simulink model "SecRwRtStBkReclnTrgtPosSelc"  (R2018b)
settings: Solver=FixedStepDiscrete  StartTime=0.0  StopTime=10.0  FixedStep=0.01  RelTol=1e-3
undefined symbols (not defined in the file or in its folder): KeSMSw4SAcsMd23SecRwRtStBkReclnUpwdDnwdPos_Val, KeSMSw4SAcsMd23SecRwRtStBkReclnUpwdDnwdPosMax_Val, KeSMSw4SAcsMd23SecRwRtStBkReclnUpwdDnwdPosMin_Val, KeSMSw4SAcsMd24SecRwRtStBkReclnUpwdDnwdPos1_Val, KeSMSw4SAcsMd24SecRwRtStBkReclnUpwdDnwdPos2_Val, KeSMSw4SAcsMd24SecRwRtStBkReclnUpwdDnwdPosMax1_Val, KeSMSw4SAcsMd24SecRwRtStBkReclnUpwdDnwdPosMax2_Val, KeSMSw4SAcsMd24SecRwRtStBkReclnUpwdDnwdPosMin1_Val, KeSMSw4SAcsMd24SecRwRtStBkReclnUpwdDnwdPosMin2_Val, KeSMSw4SAcsMd25SecRwRtStBkReclnUpwdDnwdPos_Val, KeSMSw4SAcsMd25SecRwRtStBkReclnUpwdDnwdPosMax_Val, KeSMSw4SAcsMd25SecRwRtStBkReclnUpwdDnwdPosMin_Val, KeSMSw4SAcsMd26SecRwRtStBkReclnUpwdDnwdPos_Val, KeSMSw4SAcsMd26SecRwRtStBkReclnUpwdDnwdPosMax_Val, KeSMSw4SAcsMd26SecRwRtStBkReclnUpwdDnwdPosMin_Val, KeSMSw4sLyingMDSecRwRtStBkReclnUpwdDnwdPos_Val, KeSMSw4sLyingMDSecRwRtStBkReclnUpwdDnwdPosMax_Val, KeSMSw4sLyingMDSecRwRtStBkReclnUpwdDnwdPosMin_Val, KeSMSw4sRecoveryMDSecRwRtStBkReclnUpwdDnwdPos_Val, KeSMSw4sRecoveryMDSecRwRtStBkReclnUpwdDnwdPosMax_Val, KeSMSw4sRecoveryMDSecRwRtStBkReclnUpwdDnwdPosMin_Val, KeSMSw4sVIPMDSecRwRtStBkReclnUpwdDnwdPos_Val, KeSMSw4sVIPMDSecRwRtStBkReclnUpwdDnwdPosMax_Val, KeSMSw4sVIPMDSecRwRtStBkReclnUpwdDnwdPosMin_Val, KeSMSw6sAcsEntrySecRwRtStBkReclnUpwdDnwd1Pos_Val, KeSMSw6sAcsEntrySecRwRtStBkReclnUpwdDnwdPos1Max_Val, KeSMSw6sAcsEntrySecRwRtStBkReclnUpwdDnwdPos1Min_Val, KeSMSw6sAcsEntrySecRwRtStBkReclnUpwdDnwdPos_Val, KeSMSw6sAcsEntrySecRwRtStBkReclnUpwdDnwdPosMax_Val, KeSMSw6sAcsEntrySecRwRtStBkReclnUpwdDnwdPosMin_Val, KeSMSw6sAcsExtSecRwRtStBkReclnUpwdDnwdPos_Val, KeSMSw6sAcsExtSecRwRtStBkReclnUpwdDnwdPosMax_Val, KeSMSw6sAcsExtSecRwRtStBkReclnUpwdDnwdPosMin_Val, KeSMSw6sRecoveryMdSecRwRtStBkReclnUpwdDnwdPos_Val, KeSMSw6sRecoveryMdSecRwRtStBkReclnUpwdDnwdPosMax_Val, KeSMSw6sRecoveryMdSecRwRtStBkReclnUpwdDnwdPosMin_Val, KeSMSw6sVIPSecRwRtStBkReclnUpwdDnwdPos_Val, KeSMSw6sVIPSecRwRtStBkReclnUpwdDnwdPosMax_Val, KeSMSw6sVIPSecRwRtStBkReclnUpwdDnwdPosMin_Val, KeSMSwAcsEntrySecRwRtStBkReclnUpwdDnwdPos1_Val, KeSMSwAcsEntrySecRwRtStBkReclnUpwdDnwdPos1Max_Val, KeSMSwAcsEntrySecRwRtStBkReclnUpwdDnwdPos1Min_Val, KeSMSwAcsEntrySecRwRtStBkReclnUpwdDnwdPos_Val, KeSMSwAcsEntrySecRwRtStBkReclnUpwdDnwdPosMax_Val, KeSMSwAcsEntrySecRwRtStBkReclnUpwdDnwdPosMin_Val, KeSMSwAcsExtSecRwRtStBkReclnUpwdDnwdPos_Val, KeSMSwAcsExtSecRwRtStBkReclnUpwdDnwdPosMax_Val, KeSMSwAcsExtSecRwRtStBkReclnUpwdDnwdPosMin_Val, KeSMSwAcsMd32SecRwRtStBkReclnUpwdDnwdPos1_Val, KeSMSwAcsMd32SecRwRtStBkReclnUpwdDnwdPos1Max_Val, KeSMSwAcsMd32SecRwRtStBkReclnUpwdDnwdPos1Min_Val, KeSMSwAcsMd32SecRwRtStBkReclnUpwdDnwdPos_Val, KeSMSwAcsMd32SecRwRtStBkReclnUpwdDnwdPosMax_Val, KeSMSwAcsMd32SecRwRtStBkReclnUpwdDnwdPosMin_Val, KeSMSwAcsMd53SecRwRtStBkReclnUpwdDnwdPos1_Val, KeSMSwAcsMd53SecRwRtStBkReclnUpwdDnwdPos1Max_Val, KeSMSwAcsMd53SecRwRtStBkReclnUpwdDnwdPos1Min_Val, KeSMSwAcsMd53SecRwRtStBkReclnUpwdDnwdPos_Val, KeSMSwAcsMd53SecRwRtStBkReclnUpwdDnwdPosMax_Val, KeSMSwAcsMd53SecRwRtStBkReclnUpwdDnwdPosMin_Val ... (+12)
libraries: TrgtPosSelcLib x15, simulink x2
(part 1 of 2)
settings Model: Creator=sn2xws  LastModifiedBy=sn2xws
settings Model: ModifiedHistory=|
  | 2023.8.1 V2.0.0 CR421790 增加模式21-26
  | 2023.11.7 bug 554442 便利下车max min 标定改为两套
  | 2024.5.7 V3.0.0 557 eze模式变更
  | 2024.7.8 V3.0.1 557模式流程V1.9
  | 2024.8.16 V3.0.2 靠背标定选择模块修改MD8 MD9逻辑
  | 2024 8.17 V3.0.3 md1 靠背阶段1阶段2目标位置选择逻辑变更
  | 2024.8.20 V3.0.4 md32 md53靠背选择改用CushnPos判断
settings DataIOCC: SaveFormat=StructureWithTime
settings OptimizationCC: DefaultParameterBehavior=Inlined  EnhancedBackFolding=on  PassReuseOutputArgsAs=Individual arguments  ZeroExternalMemoryAtStartup=off  ZeroInternalMemoryAtStartup=off  OptimizeBlockOrder=speed  DifferentSizesBufferReuse=on  OptimizationCustomize=off
settings DebuggingCC: ParameterTunabilityLossMsg=error
settings SFSimCC: MATLABDynamicMemAlloc=off
settings RTWCC: SystemTargetFile=autosar.tlc  GenCodeOnly=on  TemplateMakefile=ert_default_tmf  Description=AUTOSAR  GenerateReport=on  IncludeHyperlinkInReport=on  LaunchReport=on  GenerateTraceInfo=on  GenerateTraceReport=on  GenerateTraceReportSl=on  GenerateTraceReportSf=on  GenerateTraceReportEml=on  GenerateCodeMetricsReport=on
settings CodeAppCC: ForceParamTrailComments=on  IgnoreCustomStorageClasses=off  OperatorAnnotations=on  SimulinkDataObjDesc=on  SFDataObjDesc=on  InsertBlockDesc=on
settings STFCustomTargetCC: TargetLangStandard=C99 (ISO)  MultiwordLength=256  ParMdlRefBuildCompliant=on  CompOptLevelCompliant=on  IncludeMdlTerminateFcn=off  CombineOutputUpdateFcns=on  SuppressErrorStatus=on  ERTCustomFileBanners=on  SupportNonFinite=off  SupportComplex=off  SupportContinuousTime=off  SupportNonInlinedSFcns=off  RemoveResetFunc=on  MATLABClassNameForMDSCustomization=Simulink.SoftwareTarget.ERTCustomization  AutosarCompliant=on  UseToolchainInfoCompliant=on  LookupTableObjectStructAxisOrder=2,1,3,4,...  LUTObjectStructOrderEvenSpacing=Size,Table,Breakpoints  SystemTargetFile=autosar.tlc
settings ERTTargetCC: TargetLangStandard=C99 (ISO)  ConcurrentExecutionCompliant=off  IncludeMdlTerminateFcn=off  SuppressErrorStatus=on  SupportNonFinite=off  SupportComplex=off  ModelStepFunctionPrototypeControlCompliant=off  CPPClassGenCompliant=off  AutosarCompliant=on  LookupTableObjectStructAxisOrder=2,1,3,4,...  LUTObjectStructOrderEvenSpacing=Size,Table,Breakpoints  InlinedParameterPlacement=NonHierarchical  ERTCustomFileTemplate=example_file_process.tlc  ERTFilePackagingFormat=Compact

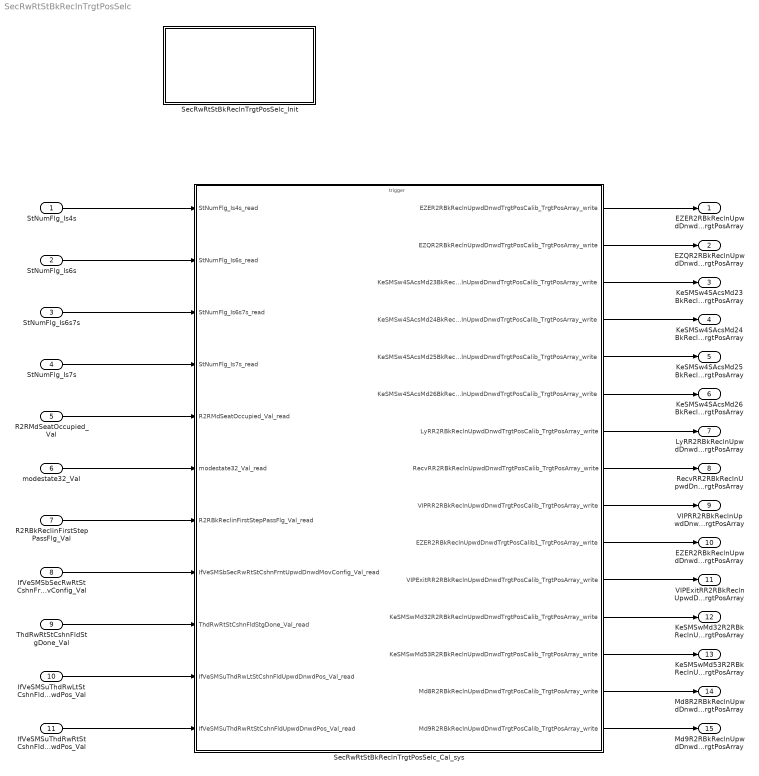
== system SecRwRtStBkReclnTrgtPosSelc ==
  StNumFlg_Is4s : Inport  OutDataTypeStr=boolean  PortDimensions=1
  StNumFlg_Is6s : Inport  Port=2  OutDataTypeStr=boolean  PortDimensions=1
  StNumFlg_Is6s7s : Inport  Port=3  OutDataTypeStr=boolean  PortDimensions=1
  StNumFlg_Is7s : Inport  Port=4  OutDataTypeStr=boolean  PortDimensions=1
  R2RMdSeatOccupied_Val : Inport  Port=5  OutDataTypeStr=boolean  PortDimensions=1
  modestate32_Val : Inport  Port=6  OutDataTypeStr=uint32  PortDimensions=1
  R2RBkReclinFirstStepPassFlg_Val : Inport  Port=7  OutDataTypeStr=boolean  PortDimensions=1
  IfVeSMSbSecRwRtStCshnFrntUpwdDnwdMovConfig_Val : Inport  Port=8  OutDataTypeStr=boolean  PortDimensions=1
  ThdRwRtStCshnFldStgDone_Val : Inport  Port=9  OutDataTypeStr=boolean  PortDimensions=1
  IfVeSMSuThdRwLtStCshnFldUpwdDnwdPos_Val : Inport  Port=10  OutDataTypeStr=uint16  PortDimensions=1
  IfVeSMSuThdRwRtStCshnFldUpwdDnwdPos_Val : Inport  Port=11  OutDataTypeStr=uint16  PortDimensions=1
  SecRwRtStBkReclnTrgtPosSelc_Cal_sys : Subsystem
  SecRwRtStBkReclnTrgtPosSelc_Init : Subsystem
  EZER2RBkReclnUpwdDnwdTrgtPosCalib_TrgtPosArray : Outport  Description=|  OutDataTypeStr=uint16  PortDimensions=3
      | 0:Pos
      | 1:Max
      | 2:Min
  EZQR2RBkReclnUpwdDnwdTrgtPosCalib_TrgtPosArray : Outport  Description=|  Port=2  OutDataTypeStr=uint16  PortDimensions=3
      | 0:Pos
      | 1:Max
      | 2:Min
  KeSMSw4SAcsMd23BkReclnUpwdDnwdTrgtPosCalib_TrgtPosArray : Outport  Description=|  Port=3  OutDataTypeStr=uint16  PortDimensions=3
      | 0:Pos
      | 1:Max
      | 2:Min
  KeSMSw4SAcsMd24BkReclnUpwdDnwdTrgtPosCalib_TrgtPosArray : Outport  Description=|  Port=4  OutDataTypeStr=uint16  PortDimensions=3
      | 0:Pos
      | 1:Max
      | 2:Min
  KeSMSw4SAcsMd25BkReclnUpwdDnwdTrgtPosCalib_TrgtPosArray : Outport  Description=|  Port=5  OutDataTypeStr=uint16  PortDimensions=3
      | 0:Pos
      | 1:Max
      | 2:Min
  KeSMSw4SAcsMd26BkReclnUpwdDnwdTrgtPosCalib_TrgtPosArray : Outport  Description=|  Port=6  OutDataTypeStr=uint16  PortDimensions=3
      | 0:Pos
      | 1:Max
      | 2:Min
  LyRR2RBkReclnUpwdDnwdTrgtPosCalib_TrgtPosArray : Outport  Description=|  Port=7  OutDataTypeStr=uint16  PortDimensions=3
      | 0:Pos
      | 1:Max
      | 2:Min
  RecvRR2RBkReclnUpwdDnwdTrgtPosCalib_TrgtPosArray : Outport  Description=|  Port=8  OutDataTypeStr=uint16  PortDimensions=3
      | 0:Pos
      | 1:Max
      | 2:Min
  VIPRR2RBkReclnUpwdDnwdTrgtPosCalib_TrgtPosArray : Outport  Description=|  Port=9  OutDataTypeStr=uint16  PortDimensions=3
      | 0:Pos
      | 1:Max
      | 2:Min
  EZER2RBkReclnUpwdDnwdTrgtPosCalib1_TrgtPosArray : Outport  Description=|  Port=10  OutDataTypeStr=uint16  PortDimensions=3
      | 0:Pos
      | 1:Max
      | 2:Min
  VIPExitRR2RBkReclnUpwdDnwdTrgtPosCalib_TrgtPosArray : Outport  Description=|  Port=11  OutDataTypeStr=uint16  PortDimensions=3
      | 0:Pos
      | 1:Max
      | 2:Min
  KeSMSwMd32R2RBkReclnUpwdDnwdTrgtPosCalib_TrgtPosArray : Outport  Description=|  Port=12  OutDataTypeStr=uint16  PortDimensions=3
      | 0:Pos
      | 1:Max
      | 2:Min
  KeSMSwMd53R2RBkReclnUpwdDnwdTrgtPosCalib_TrgtPosArray : Outport  Description=|  Port=13  OutDataTypeStr=uint16  PortDimensions=3
      | 0:Pos
      | 1:Max
      | 2:Min
  Md8R2RBkReclnUpwdDnwdTrgtPosCalib_TrgtPosArray : Outport  Description=|  Port=14  OutDataTypeStr=uint16  PortDimensions=3
      | 0:Pos
      | 1:Max
      | 2:Min
  Md9R2RBkReclnUpwdDnwdTrgtPosCalib_TrgtPosArray : Outport  Description=|  Port=15  OutDataTypeStr=uint16  PortDimensions=3
      | 0:Pos
      | 1:Max
      | 2:Min
  wires:
  StNumFlg_Is4s/1 -> SecRwRtStBkReclnTrgtPosSelc_Cal_sys/1(StNumFlg_Is4s_read)
  StNumFlg_Is6s/1 -> SecRwRtStBkReclnTrgtPosSelc_Cal_sys/2(StNumFlg_Is6s_read)
  StNumFlg_Is6s7s/1 -> SecRwRtStBkReclnTrgtPosSelc_Cal_sys/3(StNumFlg_Is6s7s_read)
  StNumFlg_Is7s/1 -> SecRwRtStBkReclnTrgtPosSelc_Cal_sys/4(StNumFlg_Is7s_read)
  SecRwRtStBkReclnTrgtPosSelc_Cal_sys/1(EZER2RBkReclnUpwdDnwdTrgtPosCalib_TrgtPosArray_write) -> EZER2RBkReclnUpwdDnwdTrgtPosCalib_TrgtPosArray/1
  SecRwRtStBkReclnTrgtPosSelc_Cal_sys/2(EZQR2RBkReclnUpwdDnwdTrgtPosCalib_TrgtPosArray_write) -> EZQR2RBkReclnUpwdDnwdTrgtPosCalib_TrgtPosArray/1
  SecRwRtStBkReclnTrgtPosSelc_Cal_sys/3(KeSMSw4SAcsMd23BkReclnUpwdDnwdTrgtPosCalib_TrgtPosArray_write) -> KeSMSw4SAcsMd23BkReclnUpwdDnwdTrgtPosCalib_TrgtPosArray/1
  SecRwRtStBkReclnTrgtPosSelc_Cal_sys/4(KeSMSw4SAcsMd24BkReclnUpwdDnwdTrgtPosCalib_TrgtPosArray_write) -> KeSMSw4SAcsMd24BkReclnUpwdDnwdTrgtPosCalib_TrgtPosArray/1
  SecRwRtStBkReclnTrgtPosSelc_Cal_sys/5(KeSMSw4SAcsMd25BkReclnUpwdDnwdTrgtPosCalib_TrgtPosArray_write) -> KeSMSw4SAcsMd25BkReclnUpwdDnwdTrgtPosCalib_TrgtPosArray/1
  SecRwRtStBkReclnTrgtPosSelc_Cal_sys/6(KeSMSw4SAcsMd26BkReclnUpwdDnwdTrgtPosCalib_TrgtPosArray_write) -> KeSMSw4SAcsMd26BkReclnUpwdDnwdTrgtPosCalib_TrgtPosArray/1
  SecRwRtStBkReclnTrgtPosSelc_Cal_sys/7(LyRR2RBkReclnUpwdDnwdTrgtPosCalib_TrgtPosArray_write) -> LyRR2RBkReclnUpwdDnwdTrgtPosCalib_TrgtPosArray/1
  SecRwRtStBkReclnTrgtPosSelc_Cal_sys/8(RecvRR2RBkReclnUpwdDnwdTrgtPosCalib_TrgtPosArray_write) -> RecvRR2RBkReclnUpwdDnwdTrgtPosCalib_TrgtPosArray/1
  SecRwRtStBkReclnTrgtPosSelc_Cal_sys/9(VIPRR2RBkReclnUpwdDnwdTrgtPosCalib_TrgtPosArray_write) -> VIPRR2RBkReclnUpwdDnwdTrgtPosCalib_TrgtPosArray/1
  R2RMdSeatOccupied_Val/1 -> SecRwRtStBkReclnTrgtPosSelc_Cal_sys/5(R2RMdSeatOccupied_Val_read)
  modestate32_Val/1 -> SecRwRtStBkReclnTrgtPosSelc_Cal_sys/6(modestate32_Val_read)
  R2RBkReclinFirstStepPassFlg_Val/1 -> SecRwRtStBkReclnTrgtPosSelc_Cal_sys/7(R2RBkReclinFirstStepPassFlg_Val_read)
  SecRwRtStBkReclnTrgtPosSelc_Cal_sys/10(EZER2RBkReclnUpwdDnwdTrgtPosCalib1_TrgtPosArray_write) -> EZER2RBkReclnUpwdDnwdTrgtPosCalib1_TrgtPosArray/1
  IfVeSMSbSecRwRtStCshnFrntUpwdDnwdMovConfig_Val/1 -> SecRwRtStBkReclnTrgtPosSelc_Cal_sys/8(IfVeSMSbSecRwRtStCshnFrntUpwdDnwdMovConfig_Val_read)
  SecRwRtStBkReclnTrgtPosSelc_Cal_sys/11(VIPExitRR2RBkReclnUpwdDnwdTrgtPosCalib_TrgtPosArray_write) -> VIPExitRR2RBkReclnUpwdDnwdTrgtPosCalib_TrgtPosArray/1
  ThdRwRtStCshnFldStgDone_Val/1 -> SecRwRtStBkReclnTrgtPosSelc_Cal_sys/9(ThdRwRtStCshnFldStgDone_Val_read)
  SecRwRtStBkReclnTrgtPosSelc_Cal_sys/12(KeSMSwMd32R2RBkReclnUpwdDnwdTrgtPosCalib_TrgtPosArray_write) -> KeSMSwMd32R2RBkReclnUpwdDnwdTrgtPosCalib_TrgtPosArray/1
  SecRwRtStBkReclnTrgtPosSelc_Cal_sys/13(KeSMSwMd53R2RBkReclnUpwdDnwdTrgtPosCalib_TrgtPosArray_write) -> KeSMSwMd53R2RBkReclnUpwdDnwdTrgtPosCalib_TrgtPosArray/1
  SecRwRtStBkReclnTrgtPosSelc_Cal_sys/14(Md8R2RBkReclnUpwdDnwdTrgtPosCalib_TrgtPosArray_write) -> Md8R2RBkReclnUpwdDnwdTrgtPosCalib_TrgtPosArray/1
  SecRwRtStBkReclnTrgtPosSelc_Cal_sys/15(Md9R2RBkReclnUpwdDnwdTrgtPosCalib_TrgtPosArray_write) -> Md9R2RBkReclnUpwdDnwdTrgtPosCalib_TrgtPosArray/1
  IfVeSMSuThdRwLtStCshnFldUpwdDnwdPos_Val/1 -> SecRwRtStBkReclnTrgtPosSelc_Cal_sys/10(IfVeSMSuThdRwLtStCshnFldUpwdDnwdPos_Val_read)
  IfVeSMSuThdRwRtStCshnFldUpwdDnwdPos_Val/1 -> SecRwRtStBkReclnTrgtPosSelc_Cal_sys/11(IfVeSMSuThdRwRtStCshnFldUpwdDnwdPos_Val_read)

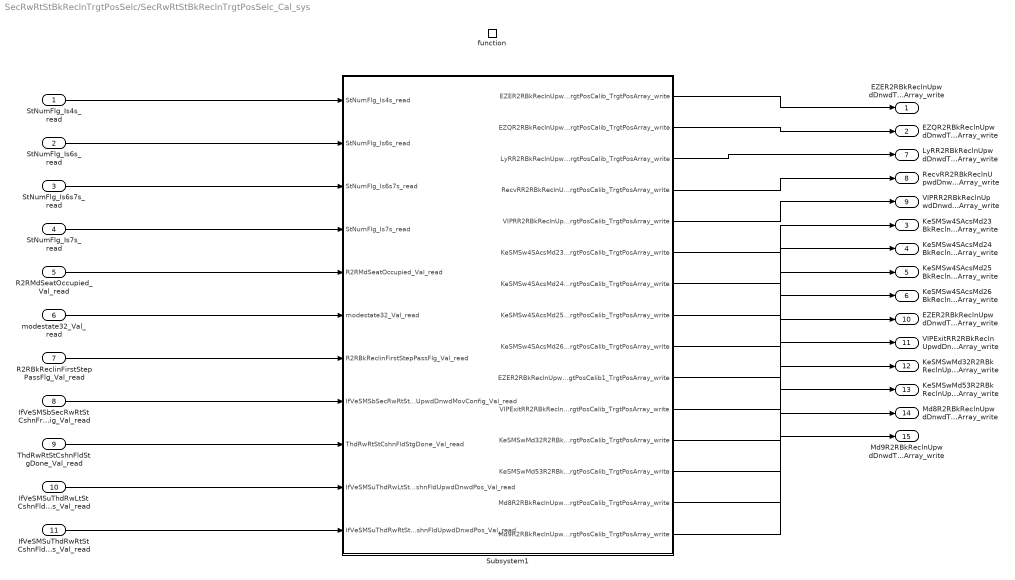
== system SecRwRtStBkReclnTrgtPosSelc/SecRwRtStBkReclnTrgtPosSelc_Cal_sys ==
  StNumFlg_Is4s_read : Inport
  StNumFlg_Is6s_read : Inport  Port=2
  StNumFlg_Is6s7s_read : Inport  Port=3
  StNumFlg_Is7s_read : Inport  Port=4
  R2RMdSeatOccupied_Val_read : Inport  Port=5
  modestate32_Val_read : Inport  Port=6
  R2RBkReclinFirstStepPassFlg_Val_read : Inport  Port=7
  IfVeSMSbSecRwRtStCshnFrntUpwdDnwdMovConfig_Val_read : Inport  Port=8
  ThdRwRtStCshnFldStgDone_Val_read : Inport  Port=9
  IfVeSMSuThdRwLtStCshnFldUpwdDnwdPos_Val_read : Inport  Port=10
  IfVeSMSuThdRwRtStCshnFldUpwdDnwdPos_Val_read : Inport  Port=11
  function : TriggerPort  TriggerType=function-call  IsSimulinkFunction=on  FunctionName=SecRwRtStBkReclnTrgtPosSelc_Cal  VariantControl=(inherit)
  Subsystem1 : Subsystem
  EZER2RBkReclnUpwdDnwdTrgtPosCalib_TrgtPosArray_write : Outport
      settings: EnsureOutportIsVirtual=on
  EZQR2RBkReclnUpwdDnwdTrgtPosCalib_TrgtPosArray_write : Outport  Port=2
      settings: EnsureOutportIsVirtual=on
  KeSMSw4SAcsMd23BkReclnUpwdDnwdTrgtPosCalib_TrgtPosArray_write : Outport  Port=3
      settings: EnsureOutportIsVirtual=on
  KeSMSw4SAcsMd24BkReclnUpwdDnwdTrgtPosCalib_TrgtPosArray_write : Outport  Port=4
      settings: EnsureOutportIsVirtual=on
  KeSMSw4SAcsMd25BkReclnUpwdDnwdTrgtPosCalib_TrgtPosArray_write : Outport  Port=5
      settings: EnsureOutportIsVirtual=on
  KeSMSw4SAcsMd26BkReclnUpwdDnwdTrgtPosCalib_TrgtPosArray_write : Outport  Port=6
      settings: EnsureOutportIsVirtual=on
  LyRR2RBkReclnUpwdDnwdTrgtPosCalib_TrgtPosArray_write : Outport  Port=7
      settings: EnsureOutportIsVirtual=on
  RecvRR2RBkReclnUpwdDnwdTrgtPosCalib_TrgtPosArray_write : Outport  Port=8
      settings: EnsureOutportIsVirtual=on
  VIPRR2RBkReclnUpwdDnwdTrgtPosCalib_TrgtPosArray_write : Outport  Port=9
      settings: EnsureOutportIsVirtual=on
  EZER2RBkReclnUpwdDnwdTrgtPosCalib1_TrgtPosArray_write : Outport  Port=10
      settings: EnsureOutportIsVirtual=on
  VIPExitRR2RBkReclnUpwdDnwdTrgtPosCalib_TrgtPosArray_write : Outport  Port=11
      settings: EnsureOutportIsVirtual=on
  KeSMSwMd32R2RBkReclnUpwdDnwdTrgtPosCalib_TrgtPosArray_write : Outport  Port=12
      settings: EnsureOutportIsVirtual=on
  KeSMSwMd53R2RBkReclnUpwdDnwdTrgtPosCalib_TrgtPosArray_write : Outport  Port=13
      settings: EnsureOutportIsVirtual=on
  Md8R2RBkReclnUpwdDnwdTrgtPosCalib_TrgtPosArray_write : Outport  Port=14
      settings: EnsureOutportIsVirtual=on
  Md9R2RBkReclnUpwdDnwdTrgtPosCalib_TrgtPosArray_write : Outport  Port=15
      settings: EnsureOutportIsVirtual=on
  wires:
  Subsystem1/3(LyRR2RBkReclnUpwdDnwdTrgtPosCalib_TrgtPosArray_write) -> LyRR2RBkReclnUpwdDnwdTrgtPosCalib_TrgtPosArray_write/1
  Subsystem1/4(RecvRR2RBkReclnUpwdDnwdTrgtPosCalib_TrgtPosArray_write) -> RecvRR2RBkReclnUpwdDnwdTrgtPosCalib_TrgtPosArray_write/1
  Subsystem1/7(KeSMSw4SAcsMd24BkReclnUpwdDnwdTrgtPosCalib_TrgtPosArray_write) -> KeSMSw4SAcsMd24BkReclnUpwdDnwdTrgtPosCalib_TrgtPosArray_write/1
  Subsystem1/8(KeSMSw4SAcsMd25BkReclnUpwdDnwdTrgtPosCalib_TrgtPosArray_write) -> KeSMSw4SAcsMd25BkReclnUpwdDnwdTrgtPosCalib_TrgtPosArray_write/1
  Subsystem1/1(EZER2RBkReclnUpwdDnwdTrgtPosCalib_TrgtPosArray_write) -> EZER2RBkReclnUpwdDnwdTrgtPosCalib_TrgtPosArray_write/1
  Subsystem1/2(EZQR2RBkReclnUpwdDnwdTrgtPosCalib_TrgtPosArray_write) -> EZQR2RBkReclnUpwdDnwdTrgtPosCalib_TrgtPosArray_write/1
  Subsystem1/5(VIPRR2RBkReclnUpwdDnwdTrgtPosCalib_TrgtPosArray_write) -> VIPRR2RBkReclnUpwdDnwdTrgtPosCalib_TrgtPosArray_write/1
  Subsystem1/6(KeSMSw4SAcsMd23BkReclnUpwdDnwdTrgtPosCalib_TrgtPosArray_write) -> KeSMSw4SAcsMd23BkReclnUpwdDnwdTrgtPosCalib_TrgtPosArray_write/1
  Subsystem1/9(KeSMSw4SAcsMd26BkReclnUpwdDnwdTrgtPosCalib_TrgtPosArray_write) -> KeSMSw4SAcsMd26BkReclnUpwdDnwdTrgtPosCalib_TrgtPosArray_write/1
  StNumFlg_Is4s_read/1 -> Subsystem1/1(StNumFlg_Is4s_read)
  StNumFlg_Is6s_read/1 -> Subsystem1/2(StNumFlg_Is6s_read)
  StNumFlg_Is6s7s_read/1 -> Subsystem1/3(StNumFlg_Is6s7s_read)
  StNumFlg_Is7s_read/1 -> Subsystem1/4(StNumFlg_Is7s_read)
  R2RMdSeatOccupied_Val_read/1 -> Subsystem1/5(R2RMdSeatOccupied_Val_read)
  Subsystem1/10(EZER2RBkReclnUpwdDnwdTrgtPosCalib1_TrgtPosArray_write) -> EZER2RBkReclnUpwdDnwdTrgtPosCalib1_TrgtPosArray_write/1
  modestate32_Val_read/1 -> Subsystem1/6(modestate32_Val_read)
  R2RBkReclinFirstStepPassFlg_Val_read/1 -> Subsystem1/7(R2RBkReclinFirstStepPassFlg_Val_read)
  Subsystem1/11(VIPExitRR2RBkReclnUpwdDnwdTrgtPosCalib_TrgtPosArray_write) -> VIPExitRR2RBkReclnUpwdDnwdTrgtPosCalib_TrgtPosArray_write/1
  IfVeSMSbSecRwRtStCshnFrntUpwdDnwdMovConfig_Val_read/1 -> Subsystem1/8(IfVeSMSbSecRwRtStCshnFrntUpwdDnwdMovConfig_Val_read)
  Subsystem1/13(KeSMSwMd53R2RBkReclnUpwdDnwdTrgtPosCalib_TrgtPosArray_write) -> KeSMSwMd53R2RBkReclnUpwdDnwdTrgtPosCalib_TrgtPosArray_write/1
  ThdRwRtStCshnFldStgDone_Val_read/1 -> Subsystem1/9(ThdRwRtStCshnFldStgDone_Val_read)
  Subsystem1/12(KeSMSwMd32R2RBkReclnUpwdDnwdTrgtPosCalib_TrgtPosArray_write) -> KeSMSwMd32R2RBkReclnUpwdDnwdTrgtPosCalib_TrgtPosArray_write/1
  Subsystem1/14(Md8R2RBkReclnUpwdDnwdTrgtPosCalib_TrgtPosArray_write) -> Md8R2RBkReclnUpwdDnwdTrgtPosCalib_TrgtPosArray_write/1
  Subsystem1/15(Md9R2RBkReclnUpwdDnwdTrgtPosCalib_TrgtPosArray_write) -> Md9R2RBkReclnUpwdDnwdTrgtPosCalib_TrgtPosArray_write/1
  IfVeSMSuThdRwLtStCshnFldUpwdDnwdPos_Val_read/1 -> Subsystem1/10(IfVeSMSuThdRwLtStCshnFldUpwdDnwdPos_Val_read)
  IfVeSMSuThdRwRtStCshnFldUpwdDnwdPos_Val_read/1 -> Subsystem1/11(IfVeSMSuThdRwRtStCshnFldUpwdDnwdPos_Val_read)

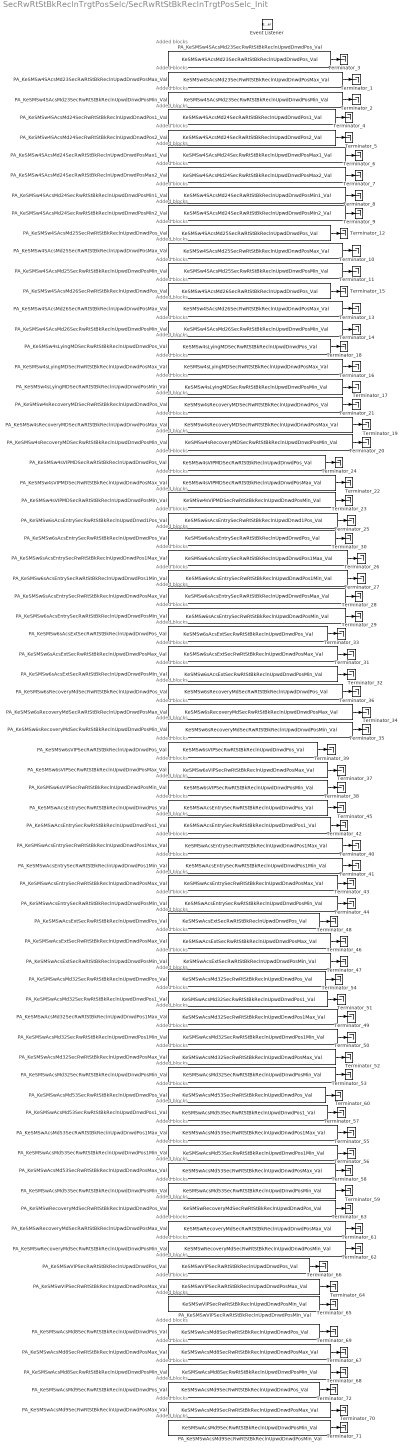
== system SecRwRtStBkReclnTrgtPosSelc/SecRwRtStBkReclnTrgtPosSelc_Init ==
  note: Added blocks
  note: Added blocks
  note: Added blocks
  note: Added blocks
  note: Added blocks
  note: Added blocks
  note: Added blocks
  note: Added blocks
  note: Added blocks
  note: Added blocks
  note: Added blocks
  note: Added blocks
  note: Added blocks
  note: Added blocks
  note: Added blocks
  note: Added blocks
  note: Added blocks
  note: Added blocks
  note: Added blocks
  note: Added blocks
  note: Added blocks
  note: Added blocks
  note: Added blocks
  note: Added blocks
  note: Added blocks
  note: Added blocks
  note: Added blocks
  note: Added blocks
  note: Added blocks
  note: Added blocks
  note: Added blocks
  note: Added blocks
  note: Added blocks
  note: Added blocks
  note: Added blocks
  note: Added blocks
  note: Added blocks
  note: Added blocks
  note: Added blocks
  note: Added blocks
  note: Added blocks
  note: Added blocks
  note: Added blocks
  note: Added blocks
  note: Added blocks
  note: Added blocks
  note: Added blocks
  note: Added blocks
  note: Added blocks
  note: Added blocks
  note: Added blocks
  note: Added blocks
  note: Added blocks
  note: Added blocks
  note: Added blocks
  note: Added blocks
  note: Added blocks
  note: Added blocks
  note: Added blocks
  note: Added blocks
  note: Added blocks
  note: Added blocks
  note: Added blocks
  note: Added blocks
  note: Added blocks
  note: Added blocks
  note: Added blocks
  note: Added blocks
  note: Added blocks
  note: Added blocks
  note: Added blocks
  note: Added blocks
  Event Listener : EventListener  EventName=reset
  PA_KeSMSw4SAcsMd23SecRwRtStBkReclnUpwdDnwdPosMax_Val : Constant  Value=KeSMSw4SAcsMd23SecRwRtStBkReclnUpwdDnwdPosMax_Val
  PA_KeSMSw4SAcsMd23SecRwRtStBkReclnUpwdDnwdPosMin_Val : Constant  Value=KeSMSw4SAcsMd23SecRwRtStBkReclnUpwdDnwdPosMin_Val
  PA_KeSMSw4SAcsMd23SecRwRtStBkReclnUpwdDnwdPos_Val : Constant  Value=KeSMSw4SAcsMd23SecRwRtStBkReclnUpwdDnwdPos_Val
  PA_KeSMSw4SAcsMd24SecRwRtStBkReclnUpwdDnwdPos1_Val : Constant  Value=KeSMSw4SAcsMd24SecRwRtStBkReclnUpwdDnwdPos1_Val
  PA_KeSMSw4SAcsMd24SecRwRtStBkReclnUpwdDnwdPos2_Val : Constant  Value=KeSMSw4SAcsMd24SecRwRtStBkReclnUpwdDnwdPos2_Val
  PA_KeSMSw4SAcsMd24SecRwRtStBkReclnUpwdDnwdPosMax1_Val : Constant  Value=KeSMSw4SAcsMd24SecRwRtStBkReclnUpwdDnwdPosMax1_Val
  PA_KeSMSw4SAcsMd24SecRwRtStBkReclnUpwdDnwdPosMax2_Val : Constant  Value=KeSMSw4SAcsMd24SecRwRtStBkReclnUpwdDnwdPosMax2_Val
  PA_KeSMSw4SAcsMd24SecRwRtStBkReclnUpwdDnwdPosMin1_Val : Constant  Value=KeSMSw4SAcsMd24SecRwRtStBkReclnUpwdDnwdPosMin1_Val
  PA_KeSMSw4SAcsMd24SecRwRtStBkReclnUpwdDnwdPosMin2_Val : Constant  Value=KeSMSw4SAcsMd24SecRwRtStBkReclnUpwdDnwdPosMin2_Val
  PA_KeSMSw4SAcsMd25SecRwRtStBkReclnUpwdDnwdPosMax_Val : Constant  Value=KeSMSw4SAcsMd25SecRwRtStBkReclnUpwdDnwdPosMax_Val
  PA_KeSMSw4SAcsMd25SecRwRtStBkReclnUpwdDnwdPosMin_Val : Constant  Value=KeSMSw4SAcsMd25SecRwRtStBkReclnUpwdDnwdPosMin_Val
  PA_KeSMSw4SAcsMd25SecRwRtStBkReclnUpwdDnwdPos_Val : Constant  Value=KeSMSw4SAcsMd25SecRwRtStBkReclnUpwdDnwdPos_Val
  PA_KeSMSw4SAcsMd26SecRwRtStBkReclnUpwdDnwdPosMax_Val : Constant  Value=KeSMSw4SAcsMd26SecRwRtStBkReclnUpwdDnwdPosMax_Val
  PA_KeSMSw4SAcsMd26SecRwRtStBkReclnUpwdDnwdPosMin_Val : Constant  Value=KeSMSw4SAcsMd26SecRwRtStBkReclnUpwdDnwdPosMin_Val
  PA_KeSMSw4SAcsMd26SecRwRtStBkReclnUpwdDnwdPos_Val : Constant  Value=KeSMSw4SAcsMd26SecRwRtStBkReclnUpwdDnwdPos_Val
  PA_KeSMSw4sLyingMDSecRwRtStBkReclnUpwdDnwdPosMax_Val : Constant  Value=KeSMSw4sLyingMDSecRwRtStBkReclnUpwdDnwdPosMax_Val
  PA_KeSMSw4sLyingMDSecRwRtStBkReclnUpwdDnwdPosMin_Val : Constant  Value=KeSMSw4sLyingMDSecRwRtStBkReclnUpwdDnwdPosMin_Val
  PA_KeSMSw4sLyingMDSecRwRtStBkReclnUpwdDnwdPos_Val : Constant  Value=KeSMSw4sLyingMDSecRwRtStBkReclnUpwdDnwdPos_Val
  PA_KeSMSw4sRecoveryMDSecRwRtStBkReclnUpwdDnwdPosMax_Val : Constant  Value=KeSMSw4sRecoveryMDSecRwRtStBkReclnUpwdDnwdPosMax_Val
  PA_KeSMSw4sRecoveryMDSecRwRtStBkReclnUpwdDnwdPosMin_Val : Constant  Value=KeSMSw4sRecoveryMDSecRwRtStBkReclnUpwdDnwdPosMin_Val
  PA_KeSMSw4sRecoveryMDSecRwRtStBkReclnUpwdDnwdPos_Val : Constant  Value=KeSMSw4sRecoveryMDSecRwRtStBkReclnUpwdDnwdPos_Val
  PA_KeSMSw4sVIPMDSecRwRtStBkReclnUpwdDnwdPosMax_Val : Constant  Value=KeSMSw4sVIPMDSecRwRtStBkReclnUpwdDnwdPosMax_Val
  PA_KeSMSw4sVIPMDSecRwRtStBkReclnUpwdDnwdPosMin_Val : Constant  Value=KeSMSw4sVIPMDSecRwRtStBkReclnUpwdDnwdPosMin_Val
  PA_KeSMSw4sVIPMDSecRwRtStBkReclnUpwdDnwdPos_Val : Constant  Value=KeSMSw4sVIPMDSecRwRtStBkReclnUpwdDnwdPos_Val
  PA_KeSMSw6sAcsEntrySecRwRtStBkReclnUpwdDnwd1Pos_Val : Constant  Value=KeSMSw6sAcsEntrySecRwRtStBkReclnUpwdDnwd1Pos_Val
  PA_KeSMSw6sAcsEntrySecRwRtStBkReclnUpwdDnwdPos1Max_Val : Constant  Value=KeSMSw6sAcsEntrySecRwRtStBkReclnUpwdDnwdPos1Max_Val
  PA_KeSMSw6sAcsEntrySecRwRtStBkReclnUpwdDnwdPos1Min_Val : Constant  Value=KeSMSw6sAcsEntrySecRwRtStBkReclnUpwdDnwdPos1Min_Val
  PA_KeSMSw6sAcsEntrySecRwRtStBkReclnUpwdDnwdPosMax_Val : Constant  Value=KeSMSw6sAcsEntrySecRwRtStBkReclnUpwdDnwdPosMax_Val
  PA_KeSMSw6sAcsEntrySecRwRtStBkReclnUpwdDnwdPosMin_Val : Constant  Value=KeSMSw6sAcsEntrySecRwRtStBkReclnUpwdDnwdPosMin_Val
  PA_KeSMSw6sAcsEntrySecRwRtStBkReclnUpwdDnwdPos_Val : Constant  Value=KeSMSw6sAcsEntrySecRwRtStBkReclnUpwdDnwdPos_Val
  PA_KeSMSw6sAcsExtSecRwRtStBkReclnUpwdDnwdPosMax_Val : Constant  Value=KeSMSw6sAcsExtSecRwRtStBkReclnUpwdDnwdPosMax_Val
  PA_KeSMSw6sAcsExtSecRwRtStBkReclnUpwdDnwdPosMin_Val : Constant  Value=KeSMSw6sAcsExtSecRwRtStBkReclnUpwdDnwdPosMin_Val
  PA_KeSMSw6sAcsExtSecRwRtStBkReclnUpwdDnwdPos_Val : Constant  Value=KeSMSw6sAcsExtSecRwRtStBkReclnUpwdDnwdPos_Val
  PA_KeSMSw6sRecoveryMdSecRwRtStBkReclnUpwdDnwdPosMax_Val : Constant  Value=KeSMSw6sRecoveryMdSecRwRtStBkReclnUpwdDnwdPosMax_Val
  PA_KeSMSw6sRecoveryMdSecRwRtStBkReclnUpwdDnwdPosMin_Val : Constant  Value=KeSMSw6sRecoveryMdSecRwRtStBkReclnUpwdDnwdPosMin_Val
  PA_KeSMSw6sRecoveryMdSecRwRtStBkReclnUpwdDnwdPos_Val : Constant  Value=KeSMSw6sRecoveryMdSecRwRtStBkReclnUpwdDnwdPos_Val
  PA_KeSMSw6sVIPSecRwRtStBkReclnUpwdDnwdPosMax_Val : Constant  Value=KeSMSw6sVIPSecRwRtStBkReclnUpwdDnwdPosMax_Val
  PA_KeSMSw6sVIPSecRwRtStBkReclnUpwdDnwdPosMin_Val : Constant  Value=KeSMSw6sVIPSecRwRtStBkReclnUpwdDnwdPosMin_Val
  PA_KeSMSw6sVIPSecRwRtStBkReclnUpwdDnwdPos_Val : Constant  Value=KeSMSw6sVIPSecRwRtStBkReclnUpwdDnwdPos_Val
  PA_KeSMSwAcsEntrySecRwRtStBkReclnUpwdDnwdPos1Max_Val : Constant  Value=KeSMSwAcsEntrySecRwRtStBkReclnUpwdDnwdPos1Max_Val
  PA_KeSMSwAcsEntrySecRwRtStBkReclnUpwdDnwdPos1Min_Val : Constant  Value=KeSMSwAcsEntrySecRwRtStBkReclnUpwdDnwdPos1Min_Val
  PA_KeSMSwAcsEntrySecRwRtStBkReclnUpwdDnwdPos1_Val : Constant  Value=KeSMSwAcsEntrySecRwRtStBkReclnUpwdDnwdPos1_Val
  PA_KeSMSwAcsEntrySecRwRtStBkReclnUpwdDnwdPosMax_Val : Constant  Value=KeSMSwAcsEntrySecRwRtStBkReclnUpwdDnwdPosMax_Val
  PA_KeSMSwAcsEntrySecRwRtStBkReclnUpwdDnwdPosMin_Val : Constant  Value=KeSMSwAcsEntrySecRwRtStBkReclnUpwdDnwdPosMin_Val
  PA_KeSMSwAcsEntrySecRwRtStBkReclnUpwdDnwdPos_Val : Constant  Value=KeSMSwAcsEntrySecRwRtStBkReclnUpwdDnwdPos_Val
  PA_KeSMSwAcsExtSecRwRtStBkReclnUpwdDnwdPosMax_Val : Constant  Value=KeSMSwAcsExtSecRwRtStBkReclnUpwdDnwdPosMax_Val
  PA_KeSMSwAcsExtSecRwRtStBkReclnUpwdDnwdPosMin_Val : Constant  Value=KeSMSwAcsExtSecRwRtStBkReclnUpwdDnwdPosMin_Val
  PA_KeSMSwAcsExtSecRwRtStBkReclnUpwdDnwdPos_Val : Constant  Value=KeSMSwAcsExtSecRwRtStBkReclnUpwdDnwdPos_Val
  PA_KeSMSwAcsMd32SecRwRtStBkReclnUpwdDnwdPos1Max_Val : Constant  Value=KeSMSwAcsMd32SecRwRtStBkReclnUpwdDnwdPos1Max_Val
  PA_KeSMSwAcsMd32SecRwRtStBkReclnUpwdDnwdPos1Min_Val : Constant  Value=KeSMSwAcsMd32SecRwRtStBkReclnUpwdDnwdPos1Min_Val
  PA_KeSMSwAcsMd32SecRwRtStBkReclnUpwdDnwdPos1_Val : Constant  Value=KeSMSwAcsMd32SecRwRtStBkReclnUpwdDnwdPos1_Val
  PA_KeSMSwAcsMd32SecRwRtStBkReclnUpwdDnwdPosMax_Val : Constant  Value=KeSMSwAcsMd32SecRwRtStBkReclnUpwdDnwdPosMax_Val
  PA_KeSMSwAcsMd32SecRwRtStBkReclnUpwdDnwdPosMin_Val : Constant  Value=KeSMSwAcsMd32SecRwRtStBkReclnUpwdDnwdPosMin_Val
  PA_KeSMSwAcsMd32SecRwRtStBkReclnUpwdDnwdPos_Val : Constant  Value=KeSMSwAcsMd32SecRwRtStBkReclnUpwdDnwdPos_Val
  PA_KeSMSwAcsMd53SecRwRtStBkReclnUpwdDnwdPos1Max_Val : Constant  Value=KeSMSwAcsMd53SecRwRtStBkReclnUpwdDnwdPos1Max_Val
  PA_KeSMSwAcsMd53SecRwRtStBkReclnUpwdDnwdPos1Min_Val : Constant  Value=KeSMSwAcsMd53SecRwRtStBkReclnUpwdDnwdPos1Min_Val
  PA_KeSMSwAcsMd53SecRwRtStBkReclnUpwdDnwdPos1_Val : Constant  Value=KeSMSwAcsMd53SecRwRtStBkReclnUpwdDnwdPos1_Val
  PA_KeSMSwAcsMd53SecRwRtStBkReclnUpwdDnwdPosMax_Val : Constant  Value=KeSMSwAcsMd53SecRwRtStBkReclnUpwdDnwdPosMax_Val
  PA_KeSMSwAcsMd53SecRwRtStBkReclnUpwdDnwdPosMin_Val : Constant  Value=KeSMSwAcsMd53SecRwRtStBkReclnUpwdDnwdPosMin_Val
  PA_KeSMSwAcsMd53SecRwRtStBkReclnUpwdDnwdPos_Val : Constant  Value=KeSMSwAcsMd53SecRwRtStBkReclnUpwdDnwdPos_Val
  PA_KeSMSwAcsMd8SecRwRtStBkReclnUpwdDnwdPosMax_Val : Constant  Value=KeSMSwAcsMd8SecRwRtStBkReclnUpwdDnwdPosMax_Val
  PA_KeSMSwAcsMd8SecRwRtStBkReclnUpwdDnwdPosMin_Val : Constant  Value=KeSMSwAcsMd8SecRwRtStBkReclnUpwdDnwdPosMin_Val
  PA_KeSMSwAcsMd8SecRwRtStBkReclnUpwdDnwdPos_Val : Constant  Value=KeSMSwAcsMd8SecRwRtStBkReclnUpwdDnwdPos_Val
  PA_KeSMSwAcsMd9SecRwRtStBkReclnUpwdDnwdPosMax_Val : Constant  Value=KeSMSwAcsMd9SecRwRtStBkReclnUpwdDnwdPosMax_Val
  PA_KeSMSwAcsMd9SecRwRtStBkReclnUpwdDnwdPosMin_Val : Constant  Value=KeSMSwAcsMd9SecRwRtStBkReclnUpwdDnwdPosMin_Val
  PA_KeSMSwAcsMd9SecRwRtStBkReclnUpwdDnwdPos_Val : Constant  Value=KeSMSwAcsMd9SecRwRtStBkReclnUpwdDnwdPos_Val
  PA_KeSMSwRecoveryMdSecRwRtStBkReclnUpwdDnwdPosMax_Val : Constant  Value=KeSMSwRecoveryMdSecRwRtStBkReclnUpwdDnwdPosMax_Val
  PA_KeSMSwRecoveryMdSecRwRtStBkReclnUpwdDnwdPosMin_Val : Constant  Value=KeSMSwRecoveryMdSecRwRtStBkReclnUpwdDnwdPosMin_Val
  PA_KeSMSwRecoveryMdSecRwRtStBkReclnUpwdDnwdPos_Val : Constant  Value=KeSMSwRecoveryMdSecRwRtStBkReclnUpwdDnwdPos_Val
  PA_KeSMSwVIPSecRwRtStBkReclnUpwdDnwdPosMax_Val : Constant  Value=KeSMSwVIPSecRwRtStBkReclnUpwdDnwdPosMax_Val
  PA_KeSMSwVIPSecRwRtStBkReclnUpwdDnwdPosMin_Val : Constant  Value=KeSMSwVIPSecRwRtStBkReclnUpwdDnwdPosMin_Val
  PA_KeSMSwVIPSecRwRtStBkReclnUpwdDnwdPos_Val : Constant  Value=KeSMSwVIPSecRwRtStBkReclnUpwdDnwdPos_Val
  Terminator_{1..72} (72 alike) : Terminator
  wires:
  PA_KeSMSw4SAcsMd23SecRwRtStBkReclnUpwdDnwdPosMax_Val/1 -> Terminator_1/1
  PA_KeSMSw4SAcsMd23SecRwRtStBkReclnUpwdDnwdPosMin_Val/1 -> Terminator_2/1
  PA_KeSMSw4SAcsMd23SecRwRtStBkReclnUpwdDnwdPos_Val/1 -> Terminator_3/1
  PA_KeSMSw4SAcsMd24SecRwRtStBkReclnUpwdDnwdPos1_Val/1 -> Terminator_4/1
  PA_KeSMSw4SAcsMd24SecRwRtStBkReclnUpwdDnwdPos2_Val/1 -> Terminator_5/1
  PA_KeSMSw4SAcsMd24SecRwRtStBkReclnUpwdDnwdPosMax1_Val/1 -> Terminator_6/1
  PA_KeSMSw4SAcsMd24SecRwRtStBkReclnUpwdDnwdPosMax2_Val/1 -> Terminator_7/1
  PA_KeSMSw4SAcsMd24SecRwRtStBkReclnUpwdDnwdPosMin1_Val/1 -> Terminator_8/1
  PA_KeSMSw4SAcsMd24SecRwRtStBkReclnUpwdDnwdPosMin2_Val/1 -> Terminator_9/1
  PA_KeSMSw4SAcsMd25SecRwRtStBkReclnUpwdDnwdPosMax_Val/1 -> Terminator_10/1
  PA_KeSMSw4SAcsMd25SecRwRtStBkReclnUpwdDnwdPosMin_Val/1 -> Terminator_11/1
  PA_KeSMSw4SAcsMd25SecRwRtStBkReclnUpwdDnwdPos_Val/1 -> Terminator_12/1
  PA_KeSMSw4SAcsMd26SecRwRtStBkReclnUpwdDnwdPosMax_Val/1 -> Terminator_13/1
  PA_KeSMSw4SAcsMd26SecRwRtStBkReclnUpwdDnwdPosMin_Val/1 -> Terminator_14/1
  PA_KeSMSw4SAcsMd26SecRwRtStBkReclnUpwdDnwdPos_Val/1 -> Terminator_15/1
  PA_KeSMSw4sLyingMDSecRwRtStBkReclnUpwdDnwdPosMax_Val/1 -> Terminator_16/1
  PA_KeSMSw4sLyingMDSecRwRtStBkReclnUpwdDnwdPosMin_Val/1 -> Terminator_17/1
  PA_KeSMSw4sLyingMDSecRwRtStBkReclnUpwdDnwdPos_Val/1 -> Terminator_18/1
  PA_KeSMSw4sRecoveryMDSecRwRtStBkReclnUpwdDnwdPosMax_Val/1 -> Terminator_19/1
  PA_KeSMSw4sRecoveryMDSecRwRtStBkReclnUpwdDnwdPosMin_Val/1 -> Terminator_20/1
  PA_KeSMSw4sRecoveryMDSecRwRtStBkReclnUpwdDnwdPos_Val/1 -> Terminator_21/1
  PA_KeSMSw4sVIPMDSecRwRtStBkReclnUpwdDnwdPosMax_Val/1 -> Terminator_22/1
  PA_KeSMSw4sVIPMDSecRwRtStBkReclnUpwdDnwdPosMin_Val/1 -> Terminator_23/1
  PA_KeSMSw4sVIPMDSecRwRtStBkReclnUpwdDnwdPos_Val/1 -> Terminator_24/1
  PA_KeSMSw6sAcsEntrySecRwRtStBkReclnUpwdDnwd1Pos_Val/1 -> Terminator_25/1
  PA_KeSMSw6sAcsEntrySecRwRtStBkReclnUpwdDnwdPos1Max_Val/1 -> Terminator_26/1
  PA_KeSMSw6sAcsEntrySecRwRtStBkReclnUpwdDnwdPos1Min_Val/1 -> Terminator_27/1
  PA_KeSMSw6sAcsEntrySecRwRtStBkReclnUpwdDnwdPosMax_Val/1 -> Terminator_28/1
  PA_KeSMSw6sAcsEntrySecRwRtStBkReclnUpwdDnwdPosMin_Val/1 -> Terminator_29/1
  PA_KeSMSw6sAcsEntrySecRwRtStBkReclnUpwdDnwdPos_Val/1 -> Terminator_30/1
  PA_KeSMSw6sAcsExtSecRwRtStBkReclnUpwdDnwdPosMax_Val/1 -> Terminator_31/1
  PA_KeSMSw6sAcsExtSecRwRtStBkReclnUpwdDnwdPosMin_Val/1 -> Terminator_32/1
  PA_KeSMSw6sAcsExtSecRwRtStBkReclnUpwdDnwdPos_Val/1 -> Terminator_33/1
  PA_KeSMSw6sRecoveryMdSecRwRtStBkReclnUpwdDnwdPosMax_Val/1 -> Terminator_34/1
  PA_KeSMSw6sRecoveryMdSecRwRtStBkReclnUpwdDnwdPosMin_Val/1 -> Terminator_35/1
  PA_KeSMSw6sRecoveryMdSecRwRtStBkReclnUpwdDnwdPos_Val/1 -> Terminator_36/1
  PA_KeSMSw6sVIPSecRwRtStBkReclnUpwdDnwdPosMax_Val/1 -> Terminator_37/1
  PA_KeSMSw6sVIPSecRwRtStBkReclnUpwdDnwdPosMin_Val/1 -> Terminator_38/1
  PA_KeSMSw6sVIPSecRwRtStBkReclnUpwdDnwdPos_Val/1 -> Terminator_39/1
  PA_KeSMSwAcsEntrySecRwRtStBkReclnUpwdDnwdPos1Max_Val/1 -> Terminator_40/1
  PA_KeSMSwAcsEntrySecRwRtStBkReclnUpwdDnwdPos1Min_Val/1 -> Terminator_41/1
  PA_KeSMSwAcsEntrySecRwRtStBkReclnUpwdDnwdPos1_Val/1 -> Terminator_42/1
  PA_KeSMSwAcsEntrySecRwRtStBkReclnUpwdDnwdPosMax_Val/1 -> Terminator_43/1
  PA_KeSMSwAcsEntrySecRwRtStBkReclnUpwdDnwdPosMin_Val/1 -> Terminator_44/1
  PA_KeSMSwAcsEntrySecRwRtStBkReclnUpwdDnwdPos_Val/1 -> Terminator_45/1
  PA_KeSMSwAcsExtSecRwRtStBkReclnUpwdDnwdPosMax_Val/1 -> Terminator_46/1
  PA_KeSMSwAcsExtSecRwRtStBkReclnUpwdDnwdPosMin_Val/1 -> Terminator_47/1
  PA_KeSMSwAcsExtSecRwRtStBkReclnUpwdDnwdPos_Val/1 -> Terminator_48/1
  PA_KeSMSwAcsMd32SecRwRtStBkReclnUpwdDnwdPos1Max_Val/1 -> Terminator_49/1
  PA_KeSMSwAcsMd32SecRwRtStBkReclnUpwdDnwdPos1Min_Val/1 -> Terminator_50/1
  PA_KeSMSwAcsMd32SecRwRtStBkReclnUpwdDnwdPos1_Val/1 -> Terminator_51/1
  PA_KeSMSwAcsMd32SecRwRtStBkReclnUpwdDnwdPosMax_Val/1 -> Terminator_52/1
  PA_KeSMSwAcsMd32SecRwRtStBkReclnUpwdDnwdPosMin_Val/1 -> Terminator_53/1
  PA_KeSMSwAcsMd32SecRwRtStBkReclnUpwdDnwdPos_Val/1 -> Terminator_54/1
  PA_KeSMSwAcsMd53SecRwRtStBkReclnUpwdDnwdPos1Max_Val/1 -> Terminator_55/1
  PA_KeSMSwAcsMd53SecRwRtStBkReclnUpwdDnwdPos1Min_Val/1 -> Terminator_56/1
  PA_KeSMSwAcsMd53SecRwRtStBkReclnUpwdDnwdPos1_Val/1 -> Terminator_57/1
  PA_KeSMSwAcsMd53SecRwRtStBkReclnUpwdDnwdPosMax_Val/1 -> Terminator_58/1
  PA_KeSMSwAcsMd53SecRwRtStBkReclnUpwdDnwdPosMin_Val/1 -> Terminator_59/1
  PA_KeSMSwAcsMd53SecRwRtStBkReclnUpwdDnwdPos_Val/1 -> Terminator_60/1
  PA_KeSMSwRecoveryMdSecRwRtStBkReclnUpwdDnwdPosMax_Val/1 -> Terminator_61/1
  PA_KeSMSwRecoveryMdSecRwRtStBkReclnUpwdDnwdPosMin_Val/1 -> Terminator_62/1
  PA_KeSMSwRecoveryMdSecRwRtStBkReclnUpwdDnwdPos_Val/1 -> Terminator_63/1
  PA_KeSMSwVIPSecRwRtStBkReclnUpwdDnwdPosMax_Val/1 -> Terminator_64/1
  PA_KeSMSwVIPSecRwRtStBkReclnUpwdDnwdPosMin_Val/1 -> Terminator_65/1
  PA_KeSMSwVIPSecRwRtStBkReclnUpwdDnwdPos_Val/1 -> Terminator_66/1
  PA_KeSMSwAcsMd8SecRwRtStBkReclnUpwdDnwdPosMax_Val/1 -> Terminator_67/1
  PA_KeSMSwAcsMd8SecRwRtStBkReclnUpwdDnwdPosMin_Val/1 -> Terminator_68/1
  PA_KeSMSwAcsMd8SecRwRtStBkReclnUpwdDnwdPos_Val/1 -> Terminator_69/1
  PA_KeSMSwAcsMd9SecRwRtStBkReclnUpwdDnwdPosMax_Val/1 -> Terminator_70/1
  PA_KeSMSwAcsMd9SecRwRtStBkReclnUpwdDnwdPosMin_Val/1 -> Terminator_71/1
  PA_KeSMSwAcsMd9SecRwRtStBkReclnUpwdDnwdPos_Val/1 -> Terminator_72/1

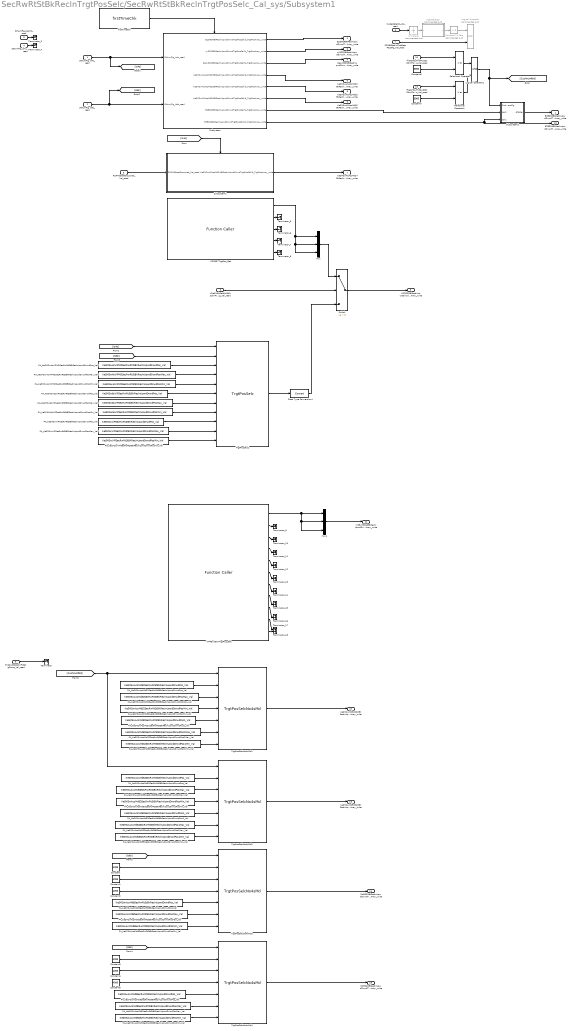
== system SecRwRtStBkReclnTrgtPosSelc/SecRwRtStBkReclnTrgtPosSelc_Cal_sys/Subsystem1 ==
  StNumFlg_Is4s_read : Inport
  StNumFlg_Is6s_read : Inport  Port=2
  StNumFlg_Is6s7s_read : Inport  Port=3
  StNumFlg_Is7s_read : Inport  Port=4
  R2RMdSeatOccupied_Val_read : Inport  Port=5
  modestate32_Val_read : Inport  Port=6
  R2RBkReclinFirstStepPassFlg_Val_read : Inport  Port=7
  IfVeSMSbSecRwRtStCshnFrntUpwdDnwdMovConfig_Val_read : Inport  Port=8
  ThdRwRtStCshnFldStgDone_Val_read : Inport  Port=9
  IfVeSMSuThdRwLtStCshnFldUpwdDnwdPos_Val_read : Inport  Port=10
  IfVeSMSuThdRwRtStCshnFldUpwdDnwdPos_Val_read : Inport  Port=11
  32BitSelector : Subsystem  Commented=on  mask(32 Bit Selector){BitNum=0}
      mask prompts: BitNum "Select Bit Number"
      mask help: Allows selection of a particular bit (0-31) out of a packed word up to 32 bits long. Output will be true if the bit number selected via the mask parameter is equal to one.
      mask TypeOptions BitNum: 0 | 1 | 2 | 3 | 4 | 5 | 6 | 7 | 8 | 9 | 10 | 11 | 12 | 13 | 14 | 15 | 16 | 17 | 18 | 19 | 20 | 21 | 22 | 23 | 24 | 25 | 26 | 27 | 28 | 29 | 30 | 31
      mask Display:
      | text(0.5, 0.8,'BIT','horizontalAlignment','center')
      | text(0.5, 0.5,'SELECTOR','horizontalAlignment','center')
      | text(0.5, 0.2,['-- Bit ',char(get_param(gcb,'BitNum')),' --'],'horizontalAlignment','center')
  Compare To Zero : simulink/Logic and Bit Operations/Compare To Zero  Commented=on  relop=>  OutDataTypeStr=boolean
  Constant{,1..5} (6 alike) : Constant  Value=4095  OutDataTypeStr=uint16
  Constant6 : Constant  Value=3960  OutDataTypeStr=uint16
  Constant7 : Constant  Value=3960  OutDataTypeStr=uint16
  Data Type Conversion4 : DataTypeConversion
  Logical Operator : Logic  Commented=on  AllPortsSameDT=off  OutDataTypeStr=boolean
  Logical Operator1 : Logic  AllPortsSameDT=off  OutDataTypeStr=boolean
  Mux : Mux  Inputs=3
  Mux1 : Mux  Inputs=3
  PA_KeSMSw4sVIPMDSecRwRtStBkReclnUpwdDnwdPosMax_Val : Constant  Value=KeSMSw4sVIPMDSecRwRtStBkReclnUpwdDnwdPosMax_Val
  PA_KeSMSw4sVIPMDSecRwRtStBkReclnUpwdDnwdPosMin_Val : Constant  Value=KeSMSw4sVIPMDSecRwRtStBkReclnUpwdDnwdPosMin_Val
  PA_KeSMSw4sVIPMDSecRwRtStBkReclnUpwdDnwdPos_Val : Constant  Value=KeSMSw4sVIPMDSecRwRtStBkReclnUpwdDnwdPos_Val
  PA_KeSMSw6sVIPSecRwRtStBkReclnUpwdDnwdPosMax_Val : Constant  Value=KeSMSw6sVIPSecRwRtStBkReclnUpwdDnwdPosMax_Val
  PA_KeSMSw6sVIPSecRwRtStBkReclnUpwdDnwdPosMin_Val : Constant  Value=KeSMSw6sVIPSecRwRtStBkReclnUpwdDnwdPosMin_Val
  PA_KeSMSw6sVIPSecRwRtStBkReclnUpwdDnwdPos_Val : Constant  Value=KeSMSw6sVIPSecRwRtStBkReclnUpwdDnwdPos_Val
  PA_KeSMSwAcsMd32SecRwRtStBkReclnUpwdDnwdPos1Max_Val : Constant  Value=KeSMSwAcsMd32SecRwRtStBkReclnUpwdDnwdPos1Max_Val
  PA_KeSMSwAcsMd32SecRwRtStBkReclnUpwdDnwdPos1Min_Val : Constant  Value=KeSMSwAcsMd32SecRwRtStBkReclnUpwdDnwdPos1Min_Val
  PA_KeSMSwAcsMd32SecRwRtStBkReclnUpwdDnwdPos1_Val : Constant  Value=KeSMSwAcsMd32SecRwRtStBkReclnUpwdDnwdPos1_Val
  PA_KeSMSwAcsMd32SecRwRtStBkReclnUpwdDnwdPosMax_Val : Constant  Value=KeSMSwAcsMd32SecRwRtStBkReclnUpwdDnwdPosMax_Val
  PA_KeSMSwAcsMd32SecRwRtStBkReclnUpwdDnwdPosMin_Val : Constant  Value=KeSMSwAcsMd32SecRwRtStBkReclnUpwdDnwdPosMin_Val
  PA_KeSMSwAcsMd32SecRwRtStBkReclnUpwdDnwdPos_Val : Constant  Value=KeSMSwAcsMd32SecRwRtStBkReclnUpwdDnwdPos_Val
  PA_KeSMSwAcsMd53SecRwRtStBkReclnUpwdDnwdPos1Max_Val : Constant  Value=KeSMSwAcsMd53SecRwRtStBkReclnUpwdDnwdPos1Max_Val
  PA_KeSMSwAcsMd53SecRwRtStBkReclnUpwdDnwdPos1Min_Val : Constant  Value=KeSMSwAcsMd53SecRwRtStBkReclnUpwdDnwdPos1Min_Val
  PA_KeSMSwAcsMd53SecRwRtStBkReclnUpwdDnwdPos1_Val : Constant  Value=KeSMSwAcsMd53SecRwRtStBkReclnUpwdDnwdPos1_Val
  PA_KeSMSwAcsMd53SecRwRtStBkReclnUpwdDnwdPosMax_Val : Constant  Value=KeSMSwAcsMd53SecRwRtStBkReclnUpwdDnwdPosMax_Val
  PA_KeSMSwAcsMd53SecRwRtStBkReclnUpwdDnwdPosMin_Val : Constant  Value=KeSMSwAcsMd53SecRwRtStBkReclnUpwdDnwdPosMin_Val
  PA_KeSMSwAcsMd53SecRwRtStBkReclnUpwdDnwdPos_Val : Constant  Value=KeSMSwAcsMd53SecRwRtStBkReclnUpwdDnwdPos_Val
  PA_KeSMSwAcsMd8SecRwRtStBkReclnUpwdDnwdPosMax_Val : Constant  Value=KeSMSwAcsMd8SecRwRtStBkReclnUpwdDnwdPosMax_Val
  PA_KeSMSwAcsMd8SecRwRtStBkReclnUpwdDnwdPosMin_Val : Constant  Value=KeSMSwAcsMd8SecRwRtStBkReclnUpwdDnwdPosMin_Val
  PA_KeSMSwAcsMd8SecRwRtStBkReclnUpwdDnwdPos_Val : Constant  Value=KeSMSwAcsMd8SecRwRtStBkReclnUpwdDnwdPos_Val
  PA_KeSMSwAcsMd9SecRwRtStBkReclnUpwdDnwdPosMax_Val : Constant  Value=KeSMSwAcsMd9SecRwRtStBkReclnUpwdDnwdPosMax_Val
  PA_KeSMSwAcsMd9SecRwRtStBkReclnUpwdDnwdPosMin_Val : Constant  Value=KeSMSwAcsMd9SecRwRtStBkReclnUpwdDnwdPosMin_Val
  PA_KeSMSwAcsMd9SecRwRtStBkReclnUpwdDnwdPos_Val : Constant  Value=KeSMSwAcsMd9SecRwRtStBkReclnUpwdDnwdPos_Val
  PA_KeSMSwVIPSecRwRtStBkReclnUpwdDnwdPosMax_Val : Constant  Value=KeSMSwVIPSecRwRtStBkReclnUpwdDnwdPosMax_Val
  PA_KeSMSwVIPSecRwRtStBkReclnUpwdDnwdPosMin_Val : Constant  Value=KeSMSwVIPSecRwRtStBkReclnUpwdDnwdPosMin_Val
  PA_KeSMSwVIPSecRwRtStBkReclnUpwdDnwdPos_Val : Constant  Value=KeSMSwVIPSecRwRtStBkReclnUpwdDnwdPos_Val
  Relational Operator : RelationalOperator  OutDataTypeStr=boolean  RndMeth=Simplest
  Relational Operator1 : RelationalOperator  OutDataTypeStr=boolean  RndMeth=Simplest
  Subsystem : Subsystem
  Subsystem1 : Subsystem
  Subsystem2 : Subsystem
  Switch : Switch  Criteria=u2 > Threshold
  Terminator : Terminator
  Terminator_{3..18} (16 alike) : Terminator
  TrgtPosSelc1 : TrgtPosSelcLib/TrgtPosSelc  SystemSampleTime=-1
  TrgtPosSelcNo4sMd{1..4} (4 alike) : TrgtPosSelcLib/TrgtPosSelcNo4sMd  SystemSampleTime=-1
  Unit Delay : UnitDelay  Commented=on  SampleTime=-1
  VIPR557TrgtPos_Get : FunctionCaller  FunctionPrototype=[SecRwLtStBkReclnTrgtPos,SecRwLtStZeroTrgtPos,SecRwLtStLgrstUpwdDnwdTrgtPos,SecRwLtStLgrstInwdOtwdTrgtPos,SecRwLtStFwdBkwdTrgtPos] = VIPR557TrgtPos_Get()  OutputArgumentSpecifications=uint16(1), uint16(1), uint16(1), uint16(1), uint16(1)
  VIPRExit557TrgtPos_Get : FunctionCaller  FunctionPrototype=[SecRwRtStBkReclnTrgtPos,SecRwRtStZeroTrgtPos,SecRwRtStLgrstUpwdDnwdTrgtPos,SecRwRtStLgrstInwdOtwdTrgtPos,ThdRwLtStBkReclnTrgtPos,ThdRwLtStFwdBkwdTrgtPos,ThdRwRtStBkReclnTrgtPos,ThdRwRtStFwdBkwdTrgtPos,PassStBkReclnTrgtPos,PassStFwdBkwdTrgtPos,SecRwRtStFwdBkwdTrgtPos] = VIPRExit557TrgtPos_Get()  OutputArgumentSpecifications=uint16(1), uint16(1), uint16(1), uint16(1), uint16(1), uint16(1), uint16(1), uint16(1), uint16(1), uint16(1), uint16(1)
  firstTimeChk : TrgtPosSelcLib/firstTimeChk  SystemSampleTime=-1
  EZER2RBkReclnUpwdDnwdTrgtPosCalib_TrgtPosArray_write : Outport
      settings: EnsureOutportIsVirtual=on
  EZQR2RBkReclnUpwdDnwdTrgtPosCalib_TrgtPosArray_write : Outport  Port=2
      settings: EnsureOutportIsVirtual=on
  LyRR2RBkReclnUpwdDnwdTrgtPosCalib_TrgtPosArray_write : Outport  Port=3
      settings: EnsureOutportIsVirtual=on
  RecvRR2RBkReclnUpwdDnwdTrgtPosCalib_TrgtPosArray_write : Outport  Port=4
      settings: EnsureOutportIsVirtual=on
  VIPRR2RBkReclnUpwdDnwdTrgtPosCalib_TrgtPosArray_write : Outport  Port=5
      settings: EnsureOutportIsVirtual=on
  KeSMSw4SAcsMd23BkReclnUpwdDnwdTrgtPosCalib_TrgtPosArray_write : Outport  Port=6
      settings: EnsureOutportIsVirtual=on
  KeSMSw4SAcsMd24BkReclnUpwdDnwdTrgtPosCalib_TrgtPosArray_write : Outport  Port=7
      settings: EnsureOutportIsVirtual=on
  KeSMSw4SAcsMd25BkReclnUpwdDnwdTrgtPosCalib_TrgtPosArray_write : Outport  Port=8
      settings: EnsureOutportIsVirtual=on
  KeSMSw4SAcsMd26BkReclnUpwdDnwdTrgtPosCalib_TrgtPosArray_write : Outport  Port=9
      settings: EnsureOutportIsVirtual=on
  EZER2RBkReclnUpwdDnwdTrgtPosCalib1_TrgtPosArray_write : Outport  Port=10
      settings: EnsureOutportIsVirtual=on
  VIPExitRR2RBkReclnUpwdDnwdTrgtPosCalib_TrgtPosArray_write : Outport  Port=11
      settings: EnsureOutportIsVirtual=on
  KeSMSwMd32R2RBkReclnUpwdDnwdTrgtPosCalib_TrgtPosArray_write : Outport  Port=12
      settings: EnsureOutportIsVirtual=on
  KeSMSwMd53R2RBkReclnUpwdDnwdTrgtPosCalib_TrgtPosArray_write : Outport  Port=13
      settings: EnsureOutportIsVirtual=on
  Md8R2RBkReclnUpwdDnwdTrgtPosCalib_TrgtPosArray_write : Outport  Port=14
      settings: EnsureOutportIsVirtual=on
  Md9R2RBkReclnUpwdDnwdTrgtPosCalib_TrgtPosArray_write : Outport  Port=15
      settings: EnsureOutportIsVirtual=on
  wires:
  Subsystem/2(LyRR2RBkReclnUpwdDnwdTrgtPosCalib_TrgtPosArray_write) -> LyRR2RBkReclnUpwdDnwdTrgtPosCalib_TrgtPosArray_write/1
  Subsystem/1(EZQR2RBkReclnUpwdDnwdTrgtPosCalib_TrgtPosArray_write) -> EZQR2RBkReclnUpwdDnwdTrgtPosCalib_TrgtPosArray_write/1
  StNumFlg_Is4s_read/1 -> [Is4s], Subsystem/1(StNumFlg_Is4s_read)
  Subsystem/3(RecvRR2RBkReclnUpwdDnwdTrgtPosCalib_TrgtPosArray_write) -> RecvRR2RBkReclnUpwdDnwdTrgtPosCalib_TrgtPosArray_write/1
  StNumFlg_Is7s_read/1 -> Terminator_4/1
  StNumFlg_Is6s7s_read/1 -> Terminator_3/1
  StNumFlg_Is6s_read/1 -> [Is6s], Subsystem/2(StNumFlg_Is6s_read)
  firstTimeChk/1 -> Subsystem/Enable
  Subsystem/4(KeSMSw4SAcsMd23BkReclnUpwdDnwdTrgtPosCalib_TrgtPosArray_write) -> KeSMSw4SAcsMd23BkReclnUpwdDnwdTrgtPosCalib_TrgtPosArray_write/1
  Subsystem/5(KeSMSw4SAcsMd25BkReclnUpwdDnwdTrgtPosCalib_TrgtPosArray_write) -> KeSMSw4SAcsMd25BkReclnUpwdDnwdTrgtPosCalib_TrgtPosArray_write/1
  Subsystem/6(KeSMSw4SAcsMd26BkReclnUpwdDnwdTrgtPosCalib_TrgtPosArray_write) -> KeSMSw4SAcsMd26BkReclnUpwdDnwdTrgtPosCalib_TrgtPosArray_write/1
  R2RMdSeatOccupied_Val_read/1 -> Subsystem1/1(R2RMdSeatOccupied_Val_read)
  Subsystem1/1(KeSMSw4SAcsMd24BkReclnUpwdDnwdTrgtPosCalib_TrgtPosArray_write) -> KeSMSw4SAcsMd24BkReclnUpwdDnwdTrgtPosCalib_TrgtPosArray_write/1
  [Is4s] -> Subsystem1/Enable
  Subsystem/8(EZER2RBkReclnUpwdDnwdTrgtPosCalib1_TrgtPosArray_write) -> EZER2RBkReclnUpwdDnwdTrgtPosCalib1_TrgtPosArray_write/1, Subsystem2/3(Cal1)
  modestate32_Val_read/1 -> Unit Delay/1
  32BitSelector/1(y) -> Compare To Zero/1
  R2RBkReclinFirstStepPassFlg_Val_read/1 -> Logical Operator/2
  Unit Delay/1 -> 32BitSelector/1(x)
  Compare To Zero/1 -> Logical Operator/1
  Subsystem2/1(EZECal) -> EZER2RBkReclnUpwdDnwdTrgtPosCalib_TrgtPosArray_write/1
  Subsystem/7(EZER2RBkReclnUpwdDnwdTrgtPosCalib_TrgtPosArray_write) -> Subsystem2/2(Cal2)
  PA_KeSMSw4sVIPMDSecRwRtStBkReclnUpwdDnwdPosMax_Val/1 -> TrgtPosSelc1/4
  PA_KeSMSwVIPSecRwRtStBkReclnUpwdDnwdPosMax_Val/1 -> TrgtPosSelc1/10
  TrgtPosSelc1/1 -> Data Type Conversion4/1
  PA_KeSMSw6sVIPSecRwRtStBkReclnUpwdDnwdPosMax_Val/1 -> TrgtPosSelc1/7
  PA_KeSMSw4sVIPMDSecRwRtStBkReclnUpwdDnwdPosMin_Val/1 -> TrgtPosSelc1/5
  PA_KeSMSwVIPSecRwRtStBkReclnUpwdDnwdPos_Val/1 -> TrgtPosSelc1/9
  [Is4s] -> TrgtPosSelc1/1
  PA_KeSMSw6sVIPSecRwRtStBkReclnUpwdDnwdPosMin_Val/1 -> TrgtPosSelc1/8
  PA_KeSMSw6sVIPSecRwRtStBkReclnUpwdDnwdPos_Val/1 -> TrgtPosSelc1/6
  [Is6s] -> TrgtPosSelc1/2
  PA_KeSMSw4sVIPMDSecRwRtStBkReclnUpwdDnwdPos_Val/1 -> TrgtPosSelc1/3
  PA_KeSMSwVIPSecRwRtStBkReclnUpwdDnwdPosMin_Val/1 -> TrgtPosSelc1/11
  IfVeSMSbSecRwRtStCshnFrntUpwdDnwdMovConfig_Val_read/1 -> Switch/2
  Data Type Conversion4/1 -> Switch/3
  Switch/1 -> VIPRR2RBkReclnUpwdDnwdTrgtPosCalib_TrgtPosArray_write/1
  Mux/1 -> Switch/1
  VIPR557TrgtPos_Get/1 -> Mux/1, Mux/2, Mux/3
  VIPRExit557TrgtPos_Get/1 -> Mux1/3, Mux1/2, Mux1/1
  Mux1/1 -> VIPExitRR2RBkReclnUpwdDnwdTrgtPosCalib_TrgtPosArray_write/1
  VIPR557TrgtPos_Get/2 -> Terminator_5/1
  VIPR557TrgtPos_Get/3 -> Terminator_6/1
  VIPR557TrgtPos_Get/4 -> Terminator_7/1
  VIPR557TrgtPos_Get/5 -> Terminator_8/1
  VIPRExit557TrgtPos_Get/2 -> Terminator_9/1
  VIPRExit557TrgtPos_Get/3 -> Terminator_10/1
  VIPRExit557TrgtPos_Get/4 -> Terminator_11/1
  VIPRExit557TrgtPos_Get/5 -> Terminator_12/1
  VIPRExit557TrgtPos_Get/6 -> Terminator_13/1
  VIPRExit557TrgtPos_Get/7 -> Terminator_14/1
  VIPRExit557TrgtPos_Get/8 -> Terminator_15/1
  VIPRExit557TrgtPos_Get/9 -> Terminator_16/1
  VIPRExit557TrgtPos_Get/10 -> Terminator_17/1
  VIPRExit557TrgtPos_Get/11 -> Terminator_18/1
  TrgtPosSelcNo4sMd1/1 -> KeSMSwMd32R2RBkReclnUpwdDnwdTrgtPosCalib_TrgtPosArray_write/1
  TrgtPosSelcNo4sMd2/1 -> KeSMSwMd53R2RBkReclnUpwdDnwdTrgtPosCalib_TrgtPosArray_write/1
  PA_KeSMSwAcsMd32SecRwRtStBkReclnUpwdDnwdPos_Val/1 -> TrgtPosSelcNo4sMd1/2
  PA_KeSMSwAcsMd32SecRwRtStBkReclnUpwdDnwdPosMax_Val/1 -> TrgtPosSelcNo4sMd1/3
  PA_KeSMSwAcsMd32SecRwRtStBkReclnUpwdDnwdPosMin_Val/1 -> TrgtPosSelcNo4sMd1/4
  PA_KeSMSwAcsMd32SecRwRtStBkReclnUpwdDnwdPos1_Val/1 -> TrgtPosSelcNo4sMd1/5
  PA_KeSMSwAcsMd32SecRwRtStBkReclnUpwdDnwdPos1Max_Val/1 -> TrgtPosSelcNo4sMd1/6
  PA_KeSMSwAcsMd32SecRwRtStBkReclnUpwdDnwdPos1Min_Val/1 -> TrgtPosSelcNo4sMd1/7
  PA_KeSMSwAcsMd53SecRwRtStBkReclnUpwdDnwdPos_Val/1 -> TrgtPosSelcNo4sMd2/2
  PA_KeSMSwAcsMd53SecRwRtStBkReclnUpwdDnwdPosMax_Val/1 -> TrgtPosSelcNo4sMd2/3
  PA_KeSMSwAcsMd53SecRwRtStBkReclnUpwdDnwdPosMin_Val/1 -> TrgtPosSelcNo4sMd2/4
  PA_KeSMSwAcsMd53SecRwRtStBkReclnUpwdDnwdPos1_Val/1 -> TrgtPosSelcNo4sMd2/5
  PA_KeSMSwAcsMd53SecRwRtStBkReclnUpwdDnwdPos1Max_Val/1 -> TrgtPosSelcNo4sMd2/6
  PA_KeSMSwAcsMd53SecRwRtStBkReclnUpwdDnwdPos1Min_Val/1 -> TrgtPosSelcNo4sMd2/7
  TrgtPosSelcNo4sMd3/1 -> Md8R2RBkReclnUpwdDnwdTrgtPosCalib_TrgtPosArray_write/1
  TrgtPosSelcNo4sMd4/1 -> Md9R2RBkReclnUpwdDnwdTrgtPosCalib_TrgtPosArray_write/1
  PA_KeSMSwAcsMd8SecRwRtStBkReclnUpwdDnwdPos_Val/1 -> TrgtPosSelcNo4sMd3/5
  PA_KeSMSwAcsMd8SecRwRtStBkReclnUpwdDnwdPosMax_Val/1 -> TrgtPosSelcNo4sMd3/6
  PA_KeSMSwAcsMd8SecRwRtStBkReclnUpwdDnwdPosMin_Val/1 -> TrgtPosSelcNo4sMd3/7
  PA_KeSMSwAcsMd9SecRwRtStBkReclnUpwdDnwdPosMin_Val/1 -> TrgtPosSelcNo4sMd4/7
  PA_KeSMSwAcsMd9SecRwRtStBkReclnUpwdDnwdPosMax_Val/1 -> TrgtPosSelcNo4sMd4/6
  PA_KeSMSwAcsMd9SecRwRtStBkReclnUpwdDnwdPos_Val/1 -> TrgtPosSelcNo4sMd4/5
  Constant/1 -> TrgtPosSelcNo4sMd3/2
  Constant1/1 -> TrgtPosSelcNo4sMd3/3
  Constant2/1 -> TrgtPosSelcNo4sMd3/4
  Constant3/1 -> TrgtPosSelcNo4sMd4/2
  Constant4/1 -> TrgtPosSelcNo4sMd4/3
  Constant5/1 -> TrgtPosSelcNo4sMd4/4
  [Is6s] -> TrgtPosSelcNo4sMd3/1
  [Is6s] -> TrgtPosSelcNo4sMd4/1
  IfVeSMSuThdRwLtStCshnFldUpwdDnwdPos_Val_read/1 -> Relational Operator/1
  Constant6/1 -> Relational Operator/2
  IfVeSMSuThdRwRtStCshnFldUpwdDnwdPos_Val_read/1 -> Relational Operator1/1
  Constant7/1 -> Relational Operator1/2
  Relational Operator/1 -> Logical Operator1/1
  Relational Operator1/1 -> Logical Operator1/2
  Logical Operator1/1 -> [CushnUnfold], Subsystem2/1(FirstStepPassFlg)
  [CushnUnfold] -> TrgtPosSelcNo4sMd2/1, TrgtPosSelcNo4sMd1/1
  ThdRwRtStCshnFldStgDone_Val_read/1 -> Terminator/1

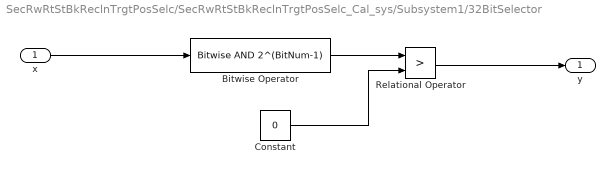
== system SecRwRtStBkReclnTrgtPosSelc/SecRwRtStBkReclnTrgtPosSelc_Cal_sys/Subsystem1/32BitSelector ==
  x : Inport
  Bitwise Operator : simulink/Logic and Bit Operations/Bitwise Operator  logicop=AND  UseBitMask=on  BitMask=2^(BitNum-1)  BitMaskRealWorld=Stored Integer
  Constant : Constant  Value=0  OutDataTypeStr=uint32
  Relational Operator : RelationalOperator  Operator=>  OutDataTypeStr=boolean  RndMeth=Simplest
  y : Outport
  wires:
  Relational Operator/1 -> y/1
  Constant/1 -> Relational Operator/2
  x/1 -> Bitwise Operator/1
  Bitwise Operator/1 -> Relational Operator/1
